simulink model "Impedance_Control"  (R2023b)
settings: Solver=VariableStepAuto  StartTime=0.0  StopTime=tf  RelTol=1e-3
values from neighbouring files (symbols this model uses):
  Bq = FindB(MassLI_Sym,MassMI_Sym,JPLi,JOLi,IntertiaLI_Sym,         IntertiaMI_Sym,TransMats,JPMi,JOMi,NumberOfJoints)    [TestFile_2.m]    (also in main.m)
undefined symbols (not defined in the file or in its folder): imp_Kd, imp_Kp
settings Model: Creator=tatwi  LastModifiedBy=danis
settings OptimizationCC: ReuseModelBlockBuffer=off

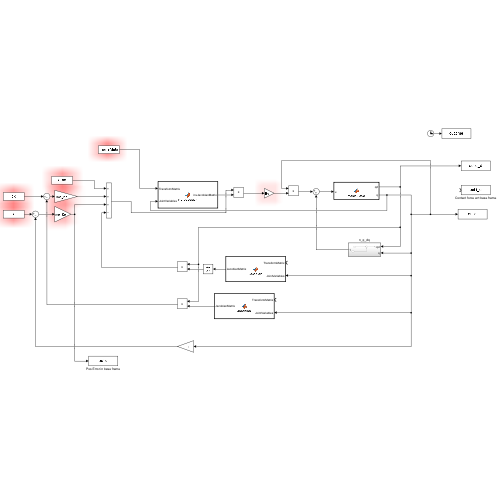
[thumbnail: Simulink's stored preview of the top-level diagram]
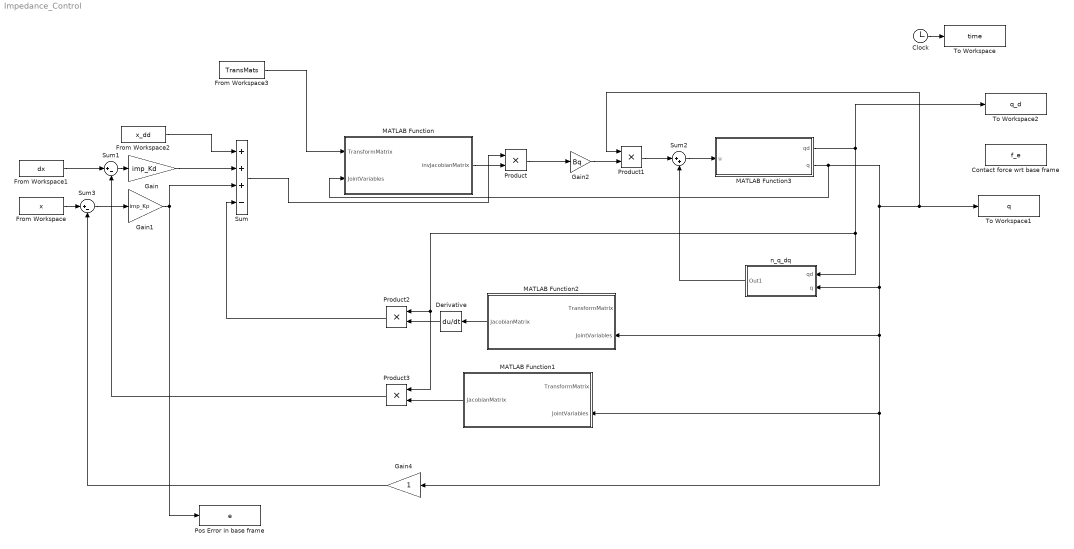
== system Impedance_Control ==
  Clock : Clock
  Contact force wrt base frame : ToWorkspace  VariableName=f_e  SaveFormat=Timeseries  SampleTime=-1
  Derivative : Derivative
  From Workspace : FromWorkspace  VariableName=x
  From Workspace1 : FromWorkspace  VariableName=dx
  From Workspace2 : FromWorkspace  VariableName=x_dd
  From Workspace3 : FromWorkspace  VariableName=TransMats
  Gain : Gain  Gain=imp_Kd
  Gain1 : Gain  Gain=imp_Kp
  Gain2 : Gain  Gain=Bq
  Gain4 : Gain
  MATLAB Function : MATLAB Function  TreatAsAtomicUnit=on
  MATLAB Function1 : MATLAB Function  TreatAsAtomicUnit=on
  MATLAB Function2 : MATLAB Function  TreatAsAtomicUnit=on
  MATLAB Function3 : MATLAB Function  TreatAsAtomicUnit=on
  Pos Error in base frame : ToWorkspace  VariableName=e  SaveFormat=Timeseries  SampleTime=-1
  Product{,1..3} (4 alike) : Product
  Sum : Sum  Inputs=+++-
  Sum1 : Sum  Inputs=|+-
  Sum2 : Sum  Inputs=|++
  Sum3 : Sum  Inputs=|+-
  To Workspace : ToWorkspace  VariableName=time  SaveFormat=Timeseries  SampleTime=-1
  To Workspace1 : ToWorkspace  VariableName=q  SaveFormat=Timeseries  SampleTime=-1
  To Workspace2 : ToWorkspace  VariableName=q_d  SaveFormat=Timeseries  SampleTime=-1
  n_q_dq : Subsystem
  wires:
  From Workspace1/1 -> Sum1/1
  From Workspace/1 -> Sum3/1
  Sum3/1 -> Gain1/1
  Sum1/1 -> Gain/1
  From Workspace2/1 -> Sum/1
  Gain1/1 -> Sum/3, Pos Error in base frame/1
  Gain/1 -> Sum/2
  Clock/1 -> To Workspace/1
  From Workspace3/1 -> MATLAB Function/1(TransformMatrix)
  n_q_dq/1(Out1) -> Sum2/2
  MATLAB Function2/1(JacobianMatrix) -> Derivative/1
  MATLAB Function/1(invJacobianMatrix) -> Product/2
  Product/1 -> Gain2/1
  Product1/1 -> Sum2/1
  Gain2/1 -> Product1/2
  Gain4/1 -> Sum3/2
  Sum2/1 -> MATLAB Function3/1(u)
  MATLAB Function3/2(q) -> n_q_dq/2(q), Gain4/1, MATLAB Function1/2(JointVariables), MATLAB Function2/2(JointVariables), Product1/1, To Workspace1/1, MATLAB Function/2(JointVariables)
  MATLAB Function3/1(qd) -> Product3/1, Product2/1, n_q_dq/1(qd), To Workspace2/1
  Derivative/1 -> Product2/2
  Product2/1 -> Sum/4
  MATLAB Function1/1(JacobianMatrix) -> Product3/2
  Product3/1 -> Sum1/2
  Sum/1 -> Product/1

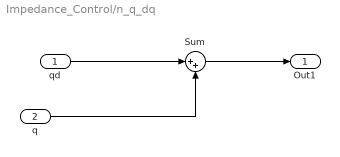
== system Impedance_Control/n_q_dq ==
  qd : Inport
  q : Inport  Port=2
  Sum : Sum  Inputs=|++
  Out1 : Outport
  wires:
  q/1 -> Sum/2
  qd/1 -> Sum/1
  Sum/1 -> Out1/1

== matlab function Impedance_Control/MATLAB Function ==
  data: TransformMatrix input; invJacobianMatrix output; JointVariables input
function invJacobianMatrix  = inv_Jacobian(TransformMatrix, JointVariables)
% NumberOfJoints = numel(JointVariables);
% position_xyz = TransformMatrix(1:3, 4);
% for i = 1:NumberOfJoints
%     JX(i) = diff(position_xyz(1), JointVariables(i));
%     JY(i) = diff(position_xyz(2), JointVariables(i));
%     JZ(i) = diff(position_xyz(3), JointVariables(i));
% end
% 
% JacobianMatrix = [JX; JY; JZ]
% invJacobianMatrix = inv(JacobianMatrix)

invJacobianMatrix = inv(jacobian([TransformMatrix(1,4),TransformMatrix(2,4),TransformMatrix(3,4)],JointVariables))

end

== matlab function Impedance_Control/MATLAB Function2 ==
  data: TransformMatrix input; JacobianMatrix output; JointVariables input
function JacobianMatrix  = Jacobian(TransformMatrix, JointVariables)
NumberOfJoints = numel(JointVariables);
position_xyz = TransformMatrix(1:3, 4);
for i = 1:NumberOfJoints
    JX(i) = diff(position_xyz(1), JointVariables(i));
    JY(i) = diff(position_xyz(2), JointVariables(i));
    JZ(i) = diff(position_xyz(3), JointVariables(i));
end

JacobianMatrix = [JX; JY; JZ];
end

== matlab function Impedance_Control/MATLAB Function3 ==
  data: qd output; u input; q output
function [qd,q]= manipulator(u)

qd = u;
q=u;

== matlab function Impedance_Control/MATLAB Function1 ==
  data: TransformMatrix input; JacobianMatrix output; JointVariables input
function JacobianMatrix  = Jacobian(TransformMatrix, JointVariables)
% NumberOfJoints = numel(JointVariables);
% position_xyz = TransformMatrix(1:3, 4);
% for i = 1:NumberOfJoints
%     JX(i) = diff(position_xyz(1), JointVariables(i));
%     JY(i) = diff(position_xyz(2), JointVariables(i));
%     JZ(i) = diff(position_xyz(3), JointVariables(i));
% end
% 
% JacobianMatrix = [JX; JY; JZ];


JacobianMatrix = jacobian([TransformMatrix(1,4),TransformMatrix(2,4),TransformMatrix(3,4)],JointVariables)

end
